simulink library "ESSLibrary"  (R2020a)
settings: Solver=VariableStepAuto  StartTime=0.0  StopTime=10.0  RelTol=1e-3
libraries: $bdroot x82, powerlib_meascontrol x10, simulink x7
(part 4 of 7)

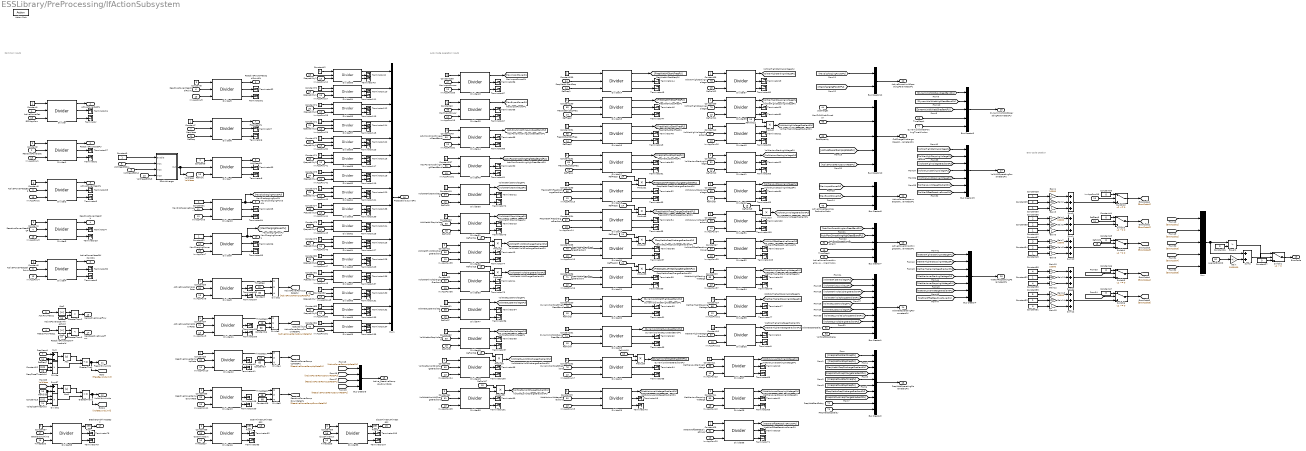
== system ESSLibrary/PreProcessing/IfActionSubsystem ==
  note: Error code creation
  note: Auto mode operation inputs
  note: Common inputs
  ActivePowerSet : Inport
  "ReactivePowerSet " : Inport  Port=2
  ActivePowerMeasECP : Inport  Port=3
  ReactivePowerMeasECP : Inport  Port=4
  ActivePowerMeasCtrlPoint : Inport  Port=5
  ReactivePowerMeasCtrlPoint : Inport  Port=6
  FreqMeas : Inport  Port=7
  VoltMeasECPL1 : Inport  Port=8
  VoltMeasECPL2 : Inport  Port=9
  VoltMeasECPL3 : Inport  Port=10
  MaxDischargingPower : Inport  Port=11
  MaxChargingPower : Inport  Port=12
  ECPAppPow : Inport  Port=13
  RefFreq : Inport  Port=14
  RefVolt : Inport  Port=15
  TimeStep : Inport  Port=16
  BreakerCmdTime : Inport  Port=17
  OpenTimeOut : Inport  Port=18
  CloseTimeOut : Inport  Port=19
  ActivePowerRampUpRate : Inport  Port=20
  ActivePowerRampDownRate : Inport  Port=21
  ReactivePowerRampUpRate : Inport  Port=22
  ReactivePowerRampDownRate : Inport  Port=23
  VoltCloseThreshold : Inport  Port=24
  FreqCloseThreshold : Inport  Port=25
  ActivePowerOpenThreshold : Inport  Port=26
  ReactivePowerOpenThreshold : Inport  Port=27
  Pcapability1 : Inport  Port=28
  Qcapability1 : Inport  Port=29
  Pcapability2 : Inport  Port=30
  Qcapability2 : Inport  Port=31
  Pcapability3 : Inport  Port=32
  Qcapability3 : Inport  Port=33
  Pcapability4 : Inport  Port=34
  Qcapability4 : Inport  Port=35
  Pcapability5 : Inport  Port=36
  Qcapability5 : Inport  Port=37
  Pcapability6 : Inport  Port=38
  Qcapability6 : Inport  Port=39
  Pcapability7 : Inport  Port=40
  Qcapability7 : Inport  Port=41
  Pcapability8 : Inport  Port=42
  Qcapability8 : Inport  Port=43
  SoCTarget : Inport  Port=44
  MaxChOrDischDuration : Inport  Port=45
  BattCapacity : Inport  Port=46
  MaxImportPower : Inport  Port=47
  MaxExportPower : Inport  Port=48
  ActivePowerReponseReductionRatio : Inport  Port=49
  ActvPowSmoothingLowDeadBand : Inport  Port=50
  ActvPowSmoothingHighDeadBand : Inport  Port=51
  ActvPowSmoothingGradient : Inport  Port=52
  ActivePowerSmoothingMovAvgTimeWindow : Inport  Port=53
  VoltWattHiStartVoltage : Inport  Port=54
  VoltWattHiStopVoltage : Inport  Port=55
  VoltWattHiVoltDischargeGradient : Inport  Port=56
  VoltWattHiVoltChargeGradient : Inport  Port=57
  VoltWattLoStartVoltage : Inport  Port=58
  VoltWattLoStopVoltage : Inport  Port=59
  VoltWattLoVoltDischargeGradient : Inport  Port=60
  VoltWattHLoVoltChargeGradient : Inport  Port=61
  VoltWattStartDelay : Inport  Port=62
  VoltWattStopDelay : Inport  Port=63
  FreqWattHiStartFreq : Inport  Port=64
  FreqWattHiStopFreq : Inport  Port=65
  FreqWattHiFreqDischargeGradient : Inport  Port=66
  FreqWattHiFreqChargeGradient : Inport  Port=67
  FreqWattLoStartFreq : Inport  Port=68
  FreqWattLoStopFreq : Inport  Port=69
  FreqWattLoFreqDischargeGradient : Inport  Port=70
  FreqWattLoFreqChargeGradient : Inport  Port=71
  FreqWattStartDelay : Inport  Port=72
  FreqWattStopDelay : Inport  Port=73
  DynamicVoltWattLowDeadBand : Inport  Port=74
  DynamicVoltWattHighDeadBand : Inport  Port=75
  DynamicVoltWattGradient : Inport  Port=76
  DynamicVoltWattMovAvgTimeWindow : Inport  Port=77
  VoltVarHighStartingVoltage : Inport  Port=78
  VoltVarHighStoppingVoltage : Inport  Port=79
  VoltVarHighVoltageGradient : Inport  Port=80
  VoltVarLowStartingVoltage : Inport  Port=81
  VoltVarLowStoppingVoltage : Inport  Port=82
  VoltVarLowVoltageGradient : Inport  Port=83
  VoltVarOffsetReactivePower : Inport  Port=84
  WattVarHighStartingWattage : Inport  Port=85
  WattVarHighStoppingWattage : Inport  Port=86
  WattVarHighWattageGradient : Inport  Port=87
  WattVarLowStartingWattage : Inport  Port=88
  WattVarLowStoppingWattage : Inport  Port=89
  WattVarLowWattageGradient : Inport  Port=90
  WattVarOffsetReactivePower : Inport  Port=91
  LogicalBlockID : Inport  Port=92  OutDataTypeStr=int32
  Action Port : ActionPort
  3PointAverge : MATLAB Function  TreatAsAtomicUnit=on
  Abs{,1..3} (4 alike) : Abs
  ActvPowMeas1 : InportShadow  Port=3
  Bus Creator1 : BusCreator  Inputs=10  OutDataTypeStr=Bus: VoltWattOperatingParametersPU
      settings: InheritFromInputs=off
  Bus Creator10 : BusCreator  Inputs=5  OutDataTypeStr=Bus: CrdChargeDischargeOperatingParametersPU
      settings: InheritFromInputs=off
  Bus Creator12 : BusCreator  Inputs=2  OutDataTypeStr=Bus: ActivePowerLimitOperatingParametersPU
      settings: InheritFromInputs=off
  Bus Creator19 : BusCreator  Inputs=7  OutDataTypeStr=Bus: VoltVarOperatingParametersPU
      settings: InheritFromInputs=off
  Bus Creator2 : BusCreator  Inputs=10  OutDataTypeStr=Bus: FreqWattOperatingParametersPU
      settings: InheritFromInputs=off
  Bus Creator3 : BusCreator  Inputs=5  OutDataTypeStr=Bus: DynamicVoltWattOperatingParameters
      settings: InheritFromInputs=off
  Bus Creator4 : BusCreator  Inputs=7  OutDataTypeStr=Bus: WattVarOperatingParametersPU
      settings: InheritFromInputs=off
  Bus Creator5 : BusCreator  Inputs=4  OutDataTypeStr=Bus: Active_ReactiveRampUp_DownData
      settings: InheritFromInputs=off
  Bus Creator7 : BusCreator  Inputs=5  OutDataTypeStr=Bus: ActivePowerSmoothingOperatingParametersPU
      settings: InheritFromInputs=off
  Bus Creator8 : BusCreator  Inputs=3  OutDataTypeStr=Bus: ActivePowerResponseOperatingParametersPU
      settings: InheritFromInputs=off
  Constant{,16..18} (4 alike) : Constant  Value=60  SampleTime=-1
  Constant{1..7,10..11,14..15,19..25,33..42,60..84,249..257,259..262,268} (67 alike) : Constant  OutDataTypeStr=boolean
  Constant12 : Constant  Value=0.01  SampleTime=-1
  Constant13 : Constant  Value=0.01  SampleTime=-1
  Constant{26..27,43..47} (7 alike) : Constant  Value=0  OutDataTypeStr=int64
  Constant{28,30,48..49,52..53} (6 alike) : Constant  OutDataTypeStr=int64
  Constant{29,54..56} (4 alike) : Constant  Value=2  OutDataTypeStr=int64
  Constant{8..9,31..32} (4 alike) : Constant  OutDataTypeStr=boolean  SampleTime=-1
  Constant50 : Constant  Value=4  OutDataTypeStr=int64
  Constant51 : Constant  Value=4  OutDataTypeStr=int64
  Constant57 : Constant  Value=3  OutDataTypeStr=int64
  Constant58 : Constant  Value=4  OutDataTypeStr=int64
  Constant59 : Constant  Value=5  OutDataTypeStr=int64
  Divide : Product  Inputs=***
  Divide1 : Product  Inputs=***
  Divide{2..5} (4 alike) : Product  Inputs=**/
  Divider{,1..69} (70 alike) : $bdroot/Divider  SystemSampleTime=-1  Latency=0  AutoFrameSizeCalculation=off
  Equal2 : RelationalOperator  Operator=>  OutDataTypeStr=boolean  RndMeth=Simplest
  Floor : Rounding  Operator=ceil
  Floor1 : Rounding  Operator=ceil
  Floor2 : Rounding  Operator=ceil
  FreqMeas1 : InportShadow  Port=7
  Gain : Gain  Gain=1000000
  Gain{1,4,7,10,13} (5 alike) : Gain  Gain=10000
  Gain{2,5,8,11,14} (5 alike) : Gain  Gain=100
  Gain{3,6,9,12,15} (5 alike) : Gain
  GreaterThan : RelationalOperator  Operator=<=  OutDataTypeStr=boolean  RndMeth=Simplest
  GreaterThan1 : RelationalOperator  Operator=<=  OutDataTypeStr=boolean  RndMeth=Simplest
  GreaterThan2 : RelationalOperator  Operator=<  OutDataTypeStr=boolean  RndMeth=Simplest
  GreaterThan3 : RelationalOperator  Operator=<  OutDataTypeStr=boolean  RndMeth=Simplest
  InvAppPow{1..51} (51 alike) : InportShadow  Port=13
  Mux : Mux  Inputs=5
  Mux1 : Mux  Inputs=16
  Product{,1..10} (11 alike) : Product
  ReactvPowMeas1 : InportShadow  Port=4
  RefFreq{1..10} (10 alike) : InportShadow  Port=14
  RefVolt{1..19} (19 alike) : InportShadow  Port=15
  Sum : Sum  Inputs=+-
  Sum{1,9..12} (5 alike) : Sum  Inputs=+++
  Sum2 : Sum  OutDataTypeStr=int64
  Sum87 : Sum  Inputs=+-
  Switch1 : Switch  Criteria=u2 > Threshold
  Switch{3..6,12} (5 alike) : Switch  Criteria=u2 ~= 0
  Terminator{,1..139} (140 alike) : Terminator
  TimeStep{1..8} (8 alike) : InportShadow  Port=16
  ActivePowerSetPU : Outport
  "ReactivePowerSetPU " : Outport  Port=2
  ActivePowerMeasPU : Outport  Port=3
  ReactivePowerMeasPU : Outport  Port=4
  ActivePowerMeasCtrlPointPU : Outport  Port=5
  ReactivePowerMeasCtrlPointPU : Outport  Port=6
  FreqMeasPU : Outport  Port=7
  VoltMeasPU : Outport  Port=8
  MaxDischargingPowerPU : Outport  Port=9
  MaxChargingPowerPU : Outport  Port=10
  FreqWithinLimits : Outport  Port=11
  VoltWithinLimits : Outport  Port=12
  ZeroActivePowerFlow : Outport  Port=13
  ZeroReactivePowerFlow : Outport  Port=14
  Active_ReactiveRampUp_DownData : Outport  Port=15  OutDataTypeStr=Bus: Active_ReactiveRampUp_DownData
  PQCapabiltyCurvePU : Outport  Port=16  OutDataTypeStr=double
  BreakerCmdTimeSteps : Outport  Port=17
  OpenTimeOutTimeSteps : Outport  Port=18
  CloseTimeOutTimeSteps : Outport  Port=19
  ActivePowerLimitOperatingParametersPU : Outport  Port=20  OutDataTypeStr=Bus: ActivePowerLimitOperatingParametersPU
  CrdChargeDischargeOperatingParametersPU : Outport  Port=21  OutDataTypeStr=Bus: CrdChargeDischargeOperatingParametersPU
  ActivePowerResponseOperatingParametersPU : Outport  Port=22  OutDataTypeStr=Bus: ActivePowerResponseOperatingParametersPU
  ActivePowerSmoothingOperatingParametersPU : Outport  Port=23  OutDataTypeStr=Bus: ActivePowerSmoothingOperatingParametersPU
  VoltWattOperatingParametersPU : Outport  Port=24  OutDataTypeStr=Bus: VoltWattOperatingParametersPU
  FreqWattOperatingParametersPU : Outport  Port=25  OutDataTypeStr=Bus: FreqWattOperatingParametersPU
  DynamicVoltWattOperatingParametersPU : Outport  Port=26  OutDataTypeStr=Bus: DynamicVoltWattOperatingParameters
  VoltVAROperatingParametersPU : Outport  Port=27  OutDataTypeStr=Bus: VoltVarOperatingParametersPU
  WattVAROperatingParametersPU : Outport  Port=28  OutDataTypeStr=Bus: WattVarOperatingParametersPU
  ErrorCode : Outport  Port=29
  tag scope: VoltMeas=global
  wires:
  VoltMeasECPL2/1 -> 3PointAverge/3(Inp2)
  VoltMeasECPL3/1 -> 3PointAverge/4(Inp3)
  RefVolt/1 -> Divider7/3
  Divider/1 -> ActivePowerSetPU/1
  Divider/3 -> Terminator/1
  Divider1/1 -> "ReactivePowerSetPU "/1
  RefFreq/1 -> Divider6/3
  InvAppPow1/1 -> Divider1/3
  InvAppPow2/1 -> Divider2/3
  InvAppPow3/1 -> Divider3/3
  Divider2/1 -> ActivePowerMeasPU/1
  Divider3/1 -> ReactivePowerMeasPU/1
  Divider4/1 -> ActivePowerMeasCtrlPointPU/1
  Divider5/1 -> ReactivePowerMeasCtrlPointPU/1
  Divider6/1 -> FreqMeasPU/1
  Divider7/1 -> VoltMeasPU/1
  [ErrorCode1] -> Mux/1
  [ErrorCode2] -> Mux/2
  [ErrorCode3] -> Mux/3
  [ErrorCode4] -> Mux/4
  [ErrorCode5] -> Mux/5
  Constant31/1 -> Divider10/1
  Constant32/1 -> Divider9/1
  MaxDischargingPower/1 -> Divider10/2
  VoltMeasECPL1/1 -> 3PointAverge/2(Inp1)
  Bus Creator5/1 -> Active_ReactiveRampUp_DownData/1
  [ActivePowerRampUpRatePU] -> Bus Creator5/1
  [ActivePowerRampDownRatePU] -> Bus Creator5/2
  [ReactivePowerRampUpRatePU] -> Bus Creator5/3
  [ReactivePowerRampDownRatePU] -> Bus Creator5/4
  Bus Creator2/1 -> FreqWattOperatingParametersPU/1
  Bus Creator3/1 -> DynamicVoltWattOperatingParametersPU/1
  Bus Creator1/1 -> VoltWattOperatingParametersPU/1
  Bus Creator7/1 -> ActivePowerSmoothingOperatingParametersPU/1
  Bus Creator8/1 -> ActivePowerResponseOperatingParametersPU/1
  Bus Creator12/1 -> ActivePowerLimitOperatingParametersPU/1
  Bus Creator10/1 -> CrdChargeDischargeOperatingParametersPU/1
  Bus Creator4/1 -> WattVAROperatingParametersPU/1
  Bus Creator19/1 -> VoltVAROperatingParametersPU/1
  InvAppPow32/1 -> Divider44/3
  Divider44/1 -> [ActvPowSmoothingLowDeadBandPU]
  Constant249/1 -> Divider44/1
  ActvPowSmoothingLowDeadBand/1 -> Divider44/2
  ActvPowSmoothingHighDeadBand/1 -> Divider45/2
  Constant257/1 -> Divider45/1
  Divider45/1 -> [ActvPowSmoothingHighDeadBandPU]
  InvAppPow31/1 -> Divider45/3
  Constant259/1 -> Divider14/1
  Divider14/1 -> [FreqWattHiStartFreqPU]
  RefFreq1/1 -> Divider14/3
  FreqWattHiStartFreq/1 -> Divider14/2
  FreqWattHiStopFreq/1 -> Divider15/2
  RefFreq2/1 -> Divider15/3
  Divider15/1 -> [FreqWattHiStopFreqPU]
  Constant250/1 -> Divider15/1
  Constant251/1 -> Divider16/1
  Divider16/1 -> [FreqWattLoStartFreqPU]
  RefFreq3/1 -> Divider16/3
  FreqWattLoStartFreq/1 -> Divider16/2
  Constant252/1 -> Divider17/1
  Divider17/1 -> [FreqWattLoStopFreqPU]
  FreqWattLoStopFreq/1 -> Divider17/2
  Constant253/1 -> Divider18/1
  InvAppPow13/1 -> Divider18/3
  FreqWattHiFreqDischargeGradient/1 -> Divider18/2
  InvAppPow14/1 -> Divider19/3
  FreqWattHiFreqChargeGradient/1 -> Divider19/2
  Constant254/1 -> Divider19/1
  FreqWattLoFreqDischargeGradient/1 -> Divider20/2
  InvAppPow15/1 -> Divider20/3
  Constant255/1 -> Divider20/1
  FreqWattLoFreqChargeGradient/1 -> Divider21/2
  InvAppPow16/1 -> Divider21/3
  Constant256/1 -> Divider21/1
  [FreqWattHiStartFreqPU] -> Bus Creator2/1
  [FreqWattHiStopFreqPU] -> Bus Creator2/2
  [FreqWattHiFreqDischargeGradientPU] -> Bus Creator2/3
  [FreqWattHiFreqChargeGradientPU] -> Bus Creator2/4
  [FreqWattLoStartFreqPU] -> Bus Creator2/5
  [FreqWattLoStopFreqPU] -> Bus Creator2/6
  [FreqWattLoFreqDischargeGradientPU] -> Bus Creator2/7
  [FreqWattLoFreqChargeGradientPU] -> Bus Creator2/8
  Constant260/1 -> Divider22/1
  RefVolt3/1 -> Divider22/3
  DynamicVoltWattHighDeadBand/1 -> Divider22/2
  Divider22/1 -> [DynamicVoltWattHighDeadBandPU]
  Divider23/1 -> [DynamicVoltWattLowDeadBandPU]
  DynamicVoltWattLowDeadBand/1 -> Divider23/2
  RefVolt4/1 -> Divider23/3
  Constant261/1 -> Divider23/1
  Constant262/1 -> Divider24/1
  InvAppPow17/1 -> Divider24/3
  DynamicVoltWattGradient/1 -> Divider24/2
  Divider30/1 -> [VoltWattHiStartVoltagePU]
  [ActvPowSmoothingLowDeadBandPU] -> Bus Creator7/1
  [ActvPowSmoothingHighDeadBandPU] -> Bus Creator7/2
  ActvPowSmoothingGradient/1 -> Bus Creator7/3
  ActivePowerSmoothingMovAvgTimeWindow/1 -> Bus Creator7/5
  Constant268/1 -> Divider43/1
  InvAppPow33/1 -> Divider43/3
  MaxImportPower/1 -> Divider43/2
  Divider43/1 -> [MaxImportPowerPU]
  [MaxImportPowerPU] -> Bus Creator8/1
  ActivePowerReponseReductionRatio/1 -> Bus Creator8/3
  SoCTarget/1 -> Bus Creator10/1
  MaxChOrDischDuration/1 -> Bus Creator10/2
  Divider10/1 -> [MaxDischargingPowerPU], MaxDischargingPowerPU/1
  Divider9/1 -> [MaxChargingPowerPU], MaxChargingPowerPU/1
  [MaxDischargingPowerPU] -> Bus Creator12/1
  [MaxChargingPowerPU] -> Bus Creator12/2
  Divider37/1 -> [VoltVarHighStartingVoltagePU]
  ECPAppPow/1 -> Divider/3
  ActivePowerRampUpRate/1 -> Divider8/2
  ActivePowerRampDownRate/1 -> Divider11/2
  ReactivePowerRampUpRate/1 -> Divider12/2
  ReactivePowerRampDownRate/1 -> Divider13/2
  Constant33/1 -> Divider8/1
  Constant34/1 -> Divider11/1
  Constant35/1 -> Divider12/1
  Constant36/1 -> Divider13/1
  ActivePowerSet/1 -> Divider/2
  "ReactivePowerSet "/1 -> Divider1/2
  Constant1/1 -> Divider/1
  Constant2/1 -> Divider1/1
  ActivePowerMeasECP/1 -> Divider2/2
  Constant3/1 -> Divider2/1
  ReactivePowerMeasECP/1 -> Divider3/2
  Constant4/1 -> Divider3/1
  ActivePowerMeasCtrlPoint/1 -> Divider4/2
  Constant5/1 -> Divider4/1
  ReactivePowerMeasCtrlPoint/1 -> Divider5/2
  Constant6/1 -> Divider5/1
  FreqMeas/1 -> Divider6/2
  Constant7/1 -> Divider6/1
  Constant8/1 -> Divider7/1
  3PointAverge/1(Out) -> Divider7/2, [VoltMeas]
  Constant9/1 -> 3PointAverge/1(Enable)
  FreqMeas1/1 -> Sum/1
  RefFreq7/1 -> Divide/1, Sum/2
  Sum/1 -> Abs/1
  GreaterThan/1 -> FreqWithinLimits/1, [FreqBeyondLimit]
  Abs/1 -> GreaterThan/1
  Divide/1 -> GreaterThan/2
  Constant12/1 -> Divide/2
  FreqCloseThreshold/1 -> Divide/3
  VoltCloseThreshold/1 -> Divide1/3
  Constant13/1 -> Divide1/2
  Divide1/1 -> GreaterThan1/2
  Abs1/1 -> GreaterThan1/1
  GreaterThan1/1 -> [VoltBeyondLimit], VoltWithinLimits/1
  Sum87/1 -> Abs1/1
  Abs2/1 -> GreaterThan2/1
  ActvPowMeas1/1 -> Abs2/1
  ActivePowerOpenThreshold/1 -> GreaterThan2/2
  ReactvPowMeas1/1 -> Abs3/1
  Abs3/1 -> GreaterThan3/1
  ReactivePowerOpenThreshold/1 -> GreaterThan3/2
  GreaterThan3/1 -> ZeroReactivePowerFlow/1
  GreaterThan2/1 -> ZeroActivePowerFlow/1
  Divide2/1 -> [ActivePowerRampUpRatePU]
  Divider8/1 -> Divide2/1
  TimeStep/1 -> Divide2/2
  Constant/1 -> Divide2/3
  TimeStep1/1 -> Divide3/2
  Constant16/1 -> Divide3/3
  Divider11/1 -> Divide3/1
  Divide3/1 -> [ActivePowerRampDownRatePU]
  Divide4/1 -> [ReactivePowerRampUpRatePU]
  Divider12/1 -> Divide4/1
  Constant17/1 -> Divide4/3
  TimeStep2/1 -> Divide4/2
  Constant18/1 -> Divide5/3
  Divider13/1 -> Divide5/1
  TimeStep3/1 -> Divide5/2
  Divide5/1 -> [ReactivePowerRampDownRatePU]
  InvAppPow36/1 -> Divider33/3
  Constant22/1 -> Divider33/1
  Divider33/2 -> Terminator14/1
  Divider32/2 -> Terminator13/1
  Constant21/1 -> Divider32/1
  InvAppPow35/1 -> Divider32/3
  Divider31/1 -> [VoltWattHiStopVoltagePU]
  RefVolt2/1 -> Divider31/3
  Constant20/1 -> Divider31/1
  Divider30/2 -> Terminator12/1
  Constant19/1 -> Divider30/1
  RefVolt1/1 -> Divider30/3
  VoltWattHiStartVoltage/1 -> Divider30/2
  VoltWattHiStopVoltage/1 -> Divider31/2
  VoltWattHiVoltDischargeGradient/1 -> Divider32/2
  VoltWattHiVoltChargeGradient/1 -> Divider33/2
  WattVarHighStoppingWattage/1 -> Divider35/2
  InvAppPow21/1 -> Divider35/3
  Constant24/1 -> Divider35/1
  Divider35/2 -> Terminator17/1
  Divider37/2 -> Terminator19/1
  Constant38/1 -> Divider37/1
  RefVolt12/1 -> Divider37/3
  WattVarHighStartingWattage/1 -> Divider34/2
  InvAppPow37/1 -> Divider34/3
  Constant23/1 -> Divider34/1
  Divider34/2 -> Terminator16/1
  Divider35/1 -> [WattVarHigherStoppingWattagePU]
  Divider34/1 -> [WattVarHigherStartingWattagePU]
  VoltVarHighStartingVoltage/1 -> Divider37/2
  InvAppPow26/1 -> Divider40/3
  Constant39/1 -> Divider39/1
  Constant40/1 -> Divider40/1
  Divider39/2 -> Terminator23/1
  RefVolt11/1 -> Divider39/3
  Divider41/2 -> Terminator22/1
  Divider39/1 -> [VoltVarHighStoppingVoltagePU]
  RefVolt10/1 -> Divider41/3
  Divider40/2 -> Terminator21/1
  Constant41/1 -> Divider41/1
  VoltVarHighStoppingVoltage/1 -> Divider39/2
  VoltVarHighVoltageGradient/1 -> Divider40/2
  VoltVarLowStartingVoltage/1 -> Divider41/2
  [DynamicVoltWattGradientPU] -> Bus Creator3/3
  TimeStep4/1 -> Bus Creator3/4
  DynamicVoltWattMovAvgTimeWindow/1 -> Bus Creator3/5
  Constant42/1 -> Divider55/1
  Gain1/1 -> Sum9/1
  Gain2/1 -> Sum9/2
  Gain3/1 -> Sum9/3
  Switch12/1 -> [ErrorCode1]
  InvAppPow38/1 -> Switch12/2
  Sum9/1 -> Switch12/3
  Constant43/1 -> Switch12/1
  Constant44/1 -> Switch3/1
  Sum1/1 -> Switch3/3
  RefFreq8/1 -> Switch3/2
  Switch3/1 -> [ErrorCode2]
  Switch4/1 -> [ErrorCode3]
  RefVolt6/1 -> Switch4/2
  Sum10/1 -> Switch4/3
  Constant45/1 -> Switch4/1
  [FreqBeyondLimit] -> Switch5/2
  Sum11/1 -> Switch5/3
  [VoltBeyondLimit] -> Switch6/2
  Sum12/1 -> Switch6/3
  Switch5/1 -> [ErrorCode4]
  Switch6/1 -> [ErrorCode5]
  Divider/2 -> Terminator24/1
  Divider1/2 -> Terminator27/1
  Divider1/3 -> Terminator2/1
  Divider2/3 -> Terminator3/1
  Divider2/2 -> Terminator28/1
  Divider3/2 -> Terminator4/1
  Divider3/3 -> Terminator29/1
  InvAppPow4/1 -> Divider4/3
  Divider4/3 -> Terminator5/1
  Divider4/2 -> Terminator30/1
  InvAppPow5/1 -> Divider5/3
  Divider6/2 -> Terminator7/1
  Divider6/3 -> Terminator6/1
  Divider5/2 -> Terminator32/1
  Divider5/3 -> Terminator31/1
  Divider7/3 -> Terminator8/1
  Divider7/2 -> Terminator33/1
  InvAppPow6/1 -> Divider10/3
  Divider10/2 -> Terminator25/1
  Divider10/3 -> Terminator34/1
  MaxChargingPower/1 -> Divider9/2
  InvAppPow7/1 -> Divider9/3
  Divider9/3 -> Terminator35/1
  Divider9/2 -> Terminator26/1
  InvAppPow8/1 -> Divider8/3
  Divider8/3 -> Terminator37/1
  Divider8/2 -> Terminator36/1
  InvAppPow9/1 -> Divider11/3
  Divider11/3 -> Terminator39/1
  Divider11/2 -> Terminator38/1
  InvAppPow10/1 -> Divider12/3
  Divider12/2 -> Terminator40/1
  Divider12/3 -> Terminator41/1
  InvAppPow11/1 -> Divider13/3
  Divider55/2 -> Terminator42/1
  Divider55/3 -> Terminator43/1
  InvAppPow12/1 -> Divider55/3
  RefFreq4/1 -> Divider17/3
  Divider31/2 -> Terminator15/1
  Sum2/1 -> Switch1/1
  Constant26/1 -> Equal2/2
  Equal2/1 -> Switch1/2
  LogicalBlockID/1 -> Gain/1
  Mux/1 -> Sum2/1, Equal2/1
  Switch1/1 -> ErrorCode/1
  Constant27/1 -> Switch1/3
  Gain/1 -> Sum2/2
  Gain6/1 -> Sum1/3
  Gain5/1 -> Sum1/2
  Gain4/1 -> Sum1/1
  Gain7/1 -> Sum10/1
  Gain8/1 -> Sum10/2
  Gain9/1 -> Sum10/3
  Gain12/1 -> Sum11/3
  Gain11/1 -> Sum11/2
  Gain10/1 -> Sum11/1
  Gain13/1 -> Sum12/1
  Gain14/1 -> Sum12/2
  Gain15/1 -> Sum12/3
  Constant28/1 -> Gain1/1
  Constant29/1 -> Gain2/1
  Constant30/1 -> Gain3/1
  Constant48/1 -> Gain6/1
  Constant49/1 -> Gain9/1
  Constant50/1 -> Gain12/1
  Constant51/1 -> Gain15/1
  Constant52/1 -> Gain11/1
  Constant53/1 -> Gain14/1
  Constant54/1 -> Gain8/1
  Constant55/1 -> Gain5/1
  Constant56/1 -> Gain4/1
  Constant57/1 -> Gain7/1
  Constant58/1 -> Gain10/1
  Constant59/1 -> Gain13/1
  Divider14/2 -> Terminator44/1
  Divider14/3 -> Terminator45/1
  Divider15/2 -> Terminator46/1
  Divider15/3 -> Terminator47/1
  Divider16/2 -> Terminator48/1
  Divider16/3 -> Terminator49/1
  Divider17/2 -> Terminator50/1
  Divider17/3 -> Terminator51/1
  Divider18/2 -> Terminator52/1
  Divider18/3 -> Terminator53/1
  Divider19/2 -> Terminator54/1
  Divider19/3 -> Terminator55/1
  Divider20/2 -> Terminator56/1
  Divider20/3 -> Terminator57/1
  Divider21/2 -> Terminator58/1
  Divider21/3 -> Terminator59/1
  Divider22/2 -> Terminator60/1
  Divider22/3 -> Terminator61/1
  Divider23/2 -> Terminator62/1
  Divider23/3 -> Terminator63/1
  Divider24/2 -> Terminator64/1
  Divider24/3 -> Terminator65/1
  Divider30/3 -> Terminator72/1
  Divider31/3 -> Terminator73/1
  Divider32/3 -> Terminator74/1
  Divider33/3 -> Terminator75/1
  Divider34/3 -> Terminator76/1
  Divider35/3 -> Terminator77/1
  Divider37/3 -> Terminator80/1
  Divider39/3 -> Terminator81/1
  Divider40/3 -> Terminator82/1
  Divider41/3 -> Terminator83/1
  Divider43/2 -> Terminator86/1
  Divider43/3 -> Terminator87/1
  Divider44/3 -> Terminator89/1
  Divider44/2 -> Terminator88/1
  Divider45/2 -> Terminator90/1
  Divider45/3 -> Terminator91/1
  RefVolt5/1 -> Divide1/1, Sum87/2
  [VoltMeas] -> Sum87/1
  FreqWattStartDelay/1 -> Bus Creator2/9
  FreqWattStopDelay/1 -> Bus Creator2/10
  [DynamicVoltWattLowDeadBandPU] -> Bus Creator3/1
  [DynamicVoltWattHighDeadBandPU] -> Bus Creator3/2
  Divider25/3 -> Terminator67/1
  Divider25/2 -> Terminator66/1
  Divider25/1 -> [MaxExportPowerPU]
  MaxExportPower/1 -> Divider25/2
  InvAppPow18/1 -> Divider25/3
  Constant60/1 -> Divider25/1
  [MaxExportPowerPU] -> Bus Creator8/2
  BattCapacity/1 -> Bus Creator10/3
  [ActivePowerRampUpRatePU] -> Bus Creator10/4
  [ActivePowerRampDownRatePU] -> Bus Creator10/5
  TimeStep5/1 -> Bus Creator7/4
  VoltWattLoStopVoltage/1 -> Divider48/2
  Divider48/2 -> Terminator95/1
  Divider48/3 -> Terminator97/1
  Constant61/1 -> Divider47/1
  Divider48/1 -> [VoltWattLoStopVoltagePU]
  Divider47/3 -> Terminator96/1
  RefVolt8/1 -> Divider48/3
  Constant62/1 -> Divider48/1
  RefVolt7/1 -> Divider47/3
  Divider47/1 -> [VoltWattLoStartVoltagePU]
  Divider47/2 -> Terminator94/1
  VoltWattLoStartVoltage/1 -> Divider47/2
  Divider50/3 -> Terminator101/1
  Divider49/3 -> Terminator100/1
  VoltWattHLoVoltChargeGradient/1 -> Divider50/2
  VoltWattLoVoltDischargeGradient/1 -> Divider49/2
  InvAppPow24/1 -> Divider49/3
  Constant63/1 -> Divider49/1
  Divider49/2 -> Terminator98/1
  Divider50/2 -> Terminator99/1
  Constant64/1 -> Divider50/1
  InvAppPow25/1 -> Divider50/3
  [VoltWattHiStartVoltagePU] -> Bus Creator1/1
  [VoltWattHiStopVoltagePU] -> Bus Creator1/2
  [VoltWattHiVoltDischargeGradientPU] -> Bus Creator1/3
  [VoltWattHiVoltChargeGradientPU] -> Bus Creator1/4
  [VoltWattLoStartVoltagePU] -> Bus Creator1/5
  [VoltWattLoStopVoltagePU] -> Bus Creator1/6
  [VoltWattLLoVoltDischargeGradientPU] -> Bus Creator1/7
  [VoltWattLoVoltChargeGradientPU] -> Bus Creator1/8
  VoltWattStartDelay/1 -> Bus Creator1/9
  VoltWattStopDelay/1 -> Bus Creator1/10
  Constant65/1 -> Divider42/1
  VoltVarLowStoppingVoltage/1 -> Divider42/2
  RefVolt9/1 -> Divider42/3
  Divider42/1 -> [VoltVarLowStoppingVoltagePU]
  Divider42/3 -> Terminator85/1
  Divider42/2 -> Terminator84/1
  Constant66/1 -> Divider51/1
  VoltVarLowVoltageGradient/1 -> Divider51/2
  InvAppPow34/1 -> Divider51/3
  Divider51/2 -> Terminator102/1
  Divider51/3 -> Terminator103/1
  Constant67/1 -> Divider52/1
  VoltVarOffsetReactivePower/1 -> Divider52/2
  InvAppPow39/1 -> Divider52/3
  Divider52/1 -> [VoltVarOffsetReactivePowerPU]
  Divider52/2 -> Terminator104/1
  Divider52/3 -> Terminator105/1
  [VoltVarOffsetReactivePowerPU] -> Bus Creator19/7
  [VoltVarLowVoltageGradientPU] -> Bus Creator19/6
  [VoltVarLowStoppingVoltagePU] -> Bus Creator19/5
  [VoltVarLowStartingVoltagePU] -> Bus Creator19/4
  [VoltVarHighVoltageGradientPU] -> Bus Creator19/3
  [VoltVarHighStoppingVoltagePU] -> Bus Creator19/2
  [VoltVarHighStartingVoltagePU] -> Bus Creator19/1
  Divider26/3 -> Terminator9/1
  Divider26/2 -> Terminator1/1
  Constant10/1 -> Divider26/1
  InvAppPow22/1 -> Divider26/3
  WattVarHighWattageGradient/1 -> Divider26/2
  Divider26/1 -> [WattVarHigherWattageGradientPU]
  Divider28/3 -> Terminator69/1
  Divider27/3 -> Terminator68/1
  Divider27/1 -> [WattVarLowerStartingWattagePU]
  Divider28/1 -> [WattVarLowerStoppingWattagePU]
  Divider27/2 -> Terminator10/1
  Constant11/1 -> Divider27/1
  Divider28/2 -> Terminator11/1
  Constant14/1 -> Divider28/1
  WattVarLowStartingWattage/1 -> Divider27/2
  WattVarLowStoppingWattage/1 -> Divider28/2
  InvAppPow23/1 -> Divider27/3
  InvAppPow40/1 -> Divider28/3
  Constant25/1 -> Divider36/1
  Divider36/2 -> Terminator20/1
  Constant15/1 -> Divider29/1
  Divider29/2 -> Terminator18/1
  Divider36/1 -> [WattVarOffsetReactivePowerPU]
  Divider29/1 -> [WattVarLowerWattageGradientPU]
  Divider29/3 -> Terminator70/1
  Divider36/3 -> Terminator71/1
  WattVarLowWattageGradient/1 -> Divider29/2
  WattVarOffsetReactivePower/1 -> Divider36/2
  InvAppPow19/1 -> Divider29/3
  InvAppPow20/1 -> Divider36/3
  [WattVarHigherStartingWattagePU] -> Bus Creator4/1
  [WattVarHigherStoppingWattagePU] -> Bus Creator4/2
  [WattVarHigherWattageGradientPU] -> Bus Creator4/3
  [WattVarLowerStartingWattagePU] -> Bus Creator4/4
  [WattVarLowerStoppingWattagePU] -> Bus Creator4/5
  [WattVarLowerWattageGradientPU] -> Bus Creator4/6
  [WattVarOffsetReactivePowerPU] -> Bus Creator4/7
  Product/1 -> [VoltVarHighVoltageGradientPU]
  Divider41/1 -> [VoltVarLowStartingVoltagePU]
  Divider40/1 -> Product/2
  RefVolt13/1 -> Product/1
  Constant46/1 -> Switch5/1
  Constant47/1 -> Switch6/1
  Divider32/1 -> Product2/2
  Product2/1 -> [VoltWattHiVoltDischargeGradientPU]
  RefVolt14/1 -> Product2/1
  Divider33/1 -> Product3/2
  Product3/1 -> [VoltWattHiVoltChargeGradientPU]
  RefVolt15/1 -> Product3/1
  Product4/1 -> [VoltWattLLoVoltDischargeGradientPU]
  Divider49/1 -> Product4/2
  RefVolt16/1 -> Product4/1
  Product5/1 -> [VoltWattLoVoltChargeGradientPU]
  Divider50/1 -> Product5/2
  RefVolt17/1 -> Product5/1
  Divider18/1 -> Product1/2
  Product1/1 -> [FreqWattHiFreqDischargeGradientPU]
  RefFreq5/1 -> Product1/1
  Divider19/1 -> Product6/2
  Product6/1 -> [FreqWattHiFreqChargeGradientPU]
  RefFreq6/1 -> Product6/1
  Divider20/1 -> Product7/2
  Product7/1 -> [FreqWattLoFreqDischargeGradientPU]
  RefFreq9/1 -> Product7/1
  Divider21/1 -> Product8/2
  Product8/1 -> [FreqWattLoFreqChargeGradientPU]
  RefFreq10/1 -> Product8/1
  Product9/1 -> [DynamicVoltWattGradientPU]
  Divider24/1 -> Product9/2
  RefVolt18/1 -> Product9/1
  Divider51/1 -> Product10/2
  Product10/1 -> [VoltVarLowVoltageGradientPU]
  RefVolt19/1 -> Product10/1
  Constant37/1 -> Divider38/1
  Constant68/1 -> Divider46/1
  Constant69/1 -> Divider53/1
  BreakerCmdTime/1 -> Divider38/2
  OpenTimeOut/1 -> Divider46/2
  CloseTimeOut/1 -> Divider53/2
  TimeStep6/1 -> Divider38/3
  TimeStep7/1 -> Divider46/3
  TimeStep8/1 -> Divider53/3
  Divider38/1 -> Floor/1
  Divider46/1 -> Floor1/1
  Divider53/1 -> Floor2/1
  Divider38/2 -> Terminator78/1
  Divider38/3 -> Terminator79/1
  Divider46/2 -> Terminator92/1
  Divider46/3 -> Terminator93/1
  Divider53/2 -> Terminator106/1
  Divider53/3 -> Terminator107/1
  Floor/1 -> BreakerCmdTimeSteps/1
  Floor1/1 -> OpenTimeOutTimeSteps/1
  Floor2/1 -> CloseTimeOutTimeSteps/1
  Divider13/2 -> Terminator108/1
  Divider13/3 -> Terminator109/1
  Pcapability1/1 -> Divider55/2
  Divider54/3 -> Terminator111/1
  Divider54/2 -> Terminator110/1
  Divider56/2 -> Terminator112/1
  Divider56/3 -> Terminator113/1
  Divider57/3 -> Terminator115/1
  Divider57/2 -> Terminator114/1
  Divider61/2 -> Terminator120/1
  Divider61/3 -> Terminator121/1
  Divider60/3 -> Terminator119/1
  Divider60/2 -> Terminator118/1
  Divider58/2 -> Terminator116/1
  Divider58/3 -> Terminator117/1
  Divider59/3 -> Terminator123/1
  Divider59/2 -> Terminator122/1
  Divider67/2 -> Terminator136/1
  Divider67/3 -> Terminator137/1
  Divider66/3 -> Terminator131/1
  Divider66/2 -> Terminator130/1
  Divider68/2 -> Terminator132/1
  Divider68/3 -> Terminator133/1
  Divider69/3 -> Terminator135/1
  Divider69/2 -> Terminator134/1
  Divider65/2 -> Terminator128/1
  Divider65/3 -> Terminator129/1
  Divider64/3 -> Terminator127/1
  Divider64/2 -> Terminator126/1
  Divider62/2 -> Terminator124/1
  Divider62/3 -> Terminator125/1
  Divider63/3 -> Terminator139/1
  Divider63/2 -> Terminator138/1
  InvAppPow27/1 -> Divider54/3
  InvAppPow28/1 -> Divider56/3
  InvAppPow29/1 -> Divider57/3
  InvAppPow30/1 -> Divider59/3
  InvAppPow41/1 -> Divider58/3
  InvAppPow42/1 -> Divider60/3
  InvAppPow43/1 -> Divider61/3
  InvAppPow44/1 -> Divider63/3
  InvAppPow45/1 -> Divider62/3
  InvAppPow46/1 -> Divider64/3
  InvAppPow47/1 -> Divider65/3
  InvAppPow48/1 -> Divider67/3
  InvAppPow49/1 -> Divider66/3
  InvAppPow50/1 -> Divider68/3
  InvAppPow51/1 -> Divider69/3
  Qcapability1/1 -> Divider54/2
  Pcapability2/1 -> Divider56/2
  Qcapability2/1 -> Divider57/2
  Pcapability3/1 -> Divider59/2
  Qcapability3/1 -> Divider58/2
  Pcapability4/1 -> Divider60/2
  Qcapability4/1 -> Divider61/2
  Pcapability5/1 -> Divider63/2
  Qcapability5/1 -> Divider62/2
  Pcapability6/1 -> Divider64/2
  Qcapability6/1 -> Divider65/2
  Pcapability7/1 -> Divider67/2
  Qcapability7/1 -> Divider66/2
  Pcapability8/1 -> Divider68/2
  Qcapability8/1 -> Divider69/2
  Constant70/1 -> Divider54/1
  Constant71/1 -> Divider56/1
  Constant72/1 -> Divider57/1
  Constant73/1 -> Divider59/1
  Constant74/1 -> Divider58/1
  Constant75/1 -> Divider60/1
  Constant76/1 -> Divider61/1
  Constant77/1 -> Divider63/1
  Constant78/1 -> Divider62/1
  Constant79/1 -> Divider64/1
  Constant80/1 -> Divider65/1
  Constant81/1 -> Divider67/1
  Constant82/1 -> Divider66/1
  Constant83/1 -> Divider68/1
  Constant84/1 -> Divider69/1
  Mux1/1 -> PQCapabiltyCurvePU/1
  Divider55/1 -> Mux1/1
  Divider69/1 -> Mux1/16
  Divider54/1 -> Mux1/2
  Divider56/1 -> Mux1/3
  Divider57/1 -> Mux1/4
  Divider59/1 -> Mux1/5
  Divider58/1 -> Mux1/6
  Divider60/1 -> Mux1/7
  Divider61/1 -> Mux1/8
  Divider63/1 -> Mux1/9
  Divider62/1 -> Mux1/10
  Divider64/1 -> Mux1/11
  Divider65/1 -> Mux1/12
  Divider67/1 -> Mux1/13
  Divider66/1 -> Mux1/14
  Divider68/1 -> Mux1/15

== system ESSLibrary/QReference_PF/If Action Subsystem ==
  PFSet : Inport
  PFSign : Inport  Port=2
  PSet : Inport  Port=3
  Action Port : ActionPort
  Subsystem1 : Subsystem
  PFSetQSet : Outport
  ErrorCode : Outport  Port=2
  wires:
  PFSign/1 -> Subsystem1/2(PFSign)
  Subsystem1/1(QOut) -> PFSetQSet/1
  PFSet/1 -> Subsystem1/1(PF)
  PSet/1 -> Subsystem1/3(PMeas)
  Subsystem1/2(ErrorCode) -> ErrorCode/1

== system ESSLibrary/QReference_PF/If Action Subsystem1 ==
  Action Port : ActionPort
  Constant : Constant  Value=0  SampleTime=-1
  PFSetQSetPU : Outport
  ErrorCode : Outport  Port=2
  wires:
  Constant/1 -> PFSetQSetPU/1, ErrorCode/1

== system ESSLibrary/SoCManagement/ElseActionSubsystem ==
  Action Port : ActionPort
  Constant1 : Constant  Value=0  OutDataTypeStr=int64  SampleTime=-1
  Constant2 : Constant  Value=0  OutDataTypeStr=boolean
  Constant3 : Constant  Value=0  OutDataTypeStr=double
  SoCFinal : Outport  OutDataTypeStr=double
  SoCNextStep : Outport  Port=2  OutDataTypeStr=double
  ChargeEnable : Outport  Port=3  OutDataTypeStr=boolean
  DischargeEnable : Outport  Port=4  OutDataTypeStr=boolean
  ErrorCodeOut : Outport  Port=5  OutDataTypeStr=int64
  wires:
  Constant2/1 -> ChargeEnable/1, DischargeEnable/1
  Constant1/1 -> ErrorCodeOut/1
  Constant3/1 -> SoCNextStep/1, SoCFinal/1

== system ESSLibrary/SoCManagement/IfActionSubsystem ==
  ActivePowerMeasECP : Inport  OutDataTypeStr=double
  SoCMeas : Inport  Port=2  OutDataTypeStr=double
  SoCMin : Inport  Port=3
  SoCMax : Inport  Port=4
  BattCapacity : Inport  Port=5  OutDataTypeStr=double
  ECPAppPow : Inport  Port=6  OutDataTypeStr=double
  TimeStep : Inport  Port=7
  ActiveReactivePowerRampUpDownData : Inport  Port=8  OutDataTypeStr=Bus: ActiveReactiveRampUpDownData
  LogicalBlockID : Inport  Port=9  OutDataTypeStr=int64
  Action Port : ActionPort
  Bus Selector : BusSelector  OutputSignals=ActivePowerRampUpRatePU,ActivePowerRampDownRatePU
  Comparator : Subsystem
  Constant1 : Constant  OutDataTypeStr=boolean
  Constant10 : Constant  Value=0  OutDataTypeStr=int64
  Constant11 : Constant  Value=0  OutDataTypeStr=int64
  Constant12 : Constant  Value=2  OutDataTypeStr=int32
  Constant13 : Constant  Value=0.0  OutDataTypeStr=double
  Constant15 : Constant  Value=0.0  OutDataTypeStr=double
  Constant17 : Constant  OutDataTypeStr=int64
  Constant5 : Constant  Value=0  OutDataTypeStr=boolean
  Constant6 : Constant  OutDataTypeStr=boolean
  Constant7 : Constant  Value=0  OutDataTypeStr=boolean
  Constant8 : Constant  OutDataTypeStr=boolean
  Equal2 : RelationalOperator  Operator=>  OutDataTypeStr=boolean  RndMeth=Simplest
  Gain1 : Gain  Gain=1000000
  RemainingEnergyCalculator : MATLAB Function  TreatAsAtomicUnit=on
  Sum1 : Sum  OutDataTypeStr=int64
  Switch : Switch  Criteria=u2 ~= 0
  Switch1 : Switch  Criteria=u2 ~= 0
  Switch4 : Switch  Criteria=u2 > Threshold
  SoCFinal : Outport  OutDataTypeStr=double
  SoCNextStep : Outport  Port=2  OutDataTypeStr=double
  ChargeEnable : Outport  Port=3
  DischargeEnable : Outport  Port=4
  ErrorCodeOut : Outport  Port=5  OutDataTypeStr=int64
  wires:
  SoCMin/1 -> Comparator/4(LowerTrhd)
  Constant1/1 -> Comparator/1(Enable/Disable)
  SoCMax/1 -> Comparator/3(UpperTrhd)
  Constant12/1 -> Comparator/5(HystSelection)
  Constant13/1 -> Comparator/7(RelHyst)
  Constant17/1 -> Comparator/8(VariableIdentifier)
  Constant15/1 -> Comparator/6(AbsHyst)
  Constant6/1 -> Switch/3
  Constant7/1 -> Switch1/1
  Constant8/1 -> Switch1/3
  Constant5/1 -> Switch/1
  SoCMeas/1 -> RemainingEnergyCalculator/2(SoCMeas)
  BattCapacity/1 -> RemainingEnergyCalculator/3(BatteryCapacity)
  ECPAppPow/1 -> RemainingEnergyCalculator/4(BasePower)
  Bus Selector/1 -> RemainingEnergyCalculator/6(ActivePowerRampUpRate)  "<ActivePowerRampUpRatePU>"
  Bus Selector/2 -> RemainingEnergyCalculator/7(ActivePowerRampDownRate)  "<ActivePowerRampDownRatePU>"
  TimeStep/1 -> RemainingEnergyCalculator/5(TimeStep)
  ActivePowerMeasECP/1 -> RemainingEnergyCalculator/1(ActivePowerMeasPU)
  Switch/1 -> ChargeEnable/1
  Switch1/1 -> DischargeEnable/1
  RemainingEnergyCalculator/1(SoCFinal) -> Comparator/2("Input "), SoCFinal/1
  RemainingEnergyCalculator/2(SoCNextStep) -> SoCNextStep/1
  Comparator/2(MaxLimitCrossed) -> Switch/2
  Comparator/3(MinLimitCrossed) -> Switch1/2
  Gain1/1 -> Sum1/2
  Equal2/1 -> Switch4/2
  Constant11/1 -> Switch4/3
  Sum1/1 -> Switch4/1
  LogicalBlockID/1 -> Gain1/1
  Switch4/1 -> ErrorCodeOut/1
  Comparator/1(ErrorCode) -> Equal2/1, Sum1/1
  Constant10/1 -> Equal2/2
  ActiveReactivePowerRampUpDownData/1 -> Bus Selector/1

== system ESSLibrary/ActivePowerSmoothing/MovAvgDeltaVoltCalc/ElseMovAvgFilter ==
  Inp : Inport
  Action Port : ActionPort
  Constant : Constant  Value=0  OutDataTypeStr=int64  SampleTime=-1
  Out : Outport
  ErrorCode : Outport  Port=2
  wires:
  Inp/1 -> Out/1
  Constant/1 -> ErrorCode/1

== system ESSLibrary/ActivePowerSmoothing/MovAvgDeltaVoltCalc/IfMovAvgFilter ==
  Inp : Inport
  FilterTime : Inport  Port=2
  TimeStep : Inport  Port=3
  Action Port : ActionPort
  Constant : Constant  Value=0
  Constant1 : Constant  Value=0
  DiscreteMovingAverage : MATLAB Function  TreatAsAtomicUnit=on
  Enabled Subsystem : Subsystem  TreatAsAtomicUnit=on
  Relational Operator : RelationalOperator  Operator=>  OutDataTypeStr=boolean  ZeroCross=off  RndMeth=Simplest
  Switch : Switch  Criteria=u2 > Threshold
  Out : Outport
  ErrorCode : Outport  Port=2
  wires:
  Inp/1 -> DiscreteMovingAverage/2(Inp)
  Constant/1 -> Relational Operator/2
  FilterTime/1 -> Enabled Subsystem/2(FilterTime)
  Switch/1 -> DiscreteMovingAverage/1(NoOfTS)
  Enabled Subsystem/1(NoOfTimeStep) -> Switch/1
  Relational Operator/1 -> Switch/2, Enabled Subsystem/Enable
  TimeStep/1 -> Enabled Subsystem/1(TimeStep), Relational Operator/1
  DiscreteMovingAverage/1(Out) -> Out/1
  Constant1/1 -> Switch/3
  DiscreteMovingAverage/2(ErrorCode) -> ErrorCode/1

== system ESSLibrary/ChargeDischargeStorageMode/Comparator/Basic alarm ver2.0 ==
  Enable/disable : Inport  OutDataTypeStr=boolean
  "Input " : Inport  Port=2
  UpperTrhd : Inport  Port=3
  LowerTrhd : Inport  Port=4
  HystSelection : Inport  Port=5  OutDataTypeStr=int32
  AbsHyst : Inport  Port=6
  RelHyst : Inport  Port=7
  Enable/disable1 : InportShadow  OutDataTypeStr=boolean
  Enabled Subsystem : Subsystem  TreatAsAtomicUnit=on
  Enabled Subsystem1 : Subsystem  TreatAsAtomicUnit=on
  If : If  IfExpression=u1 ~=0
  Switch : Switch  Criteria=u2 > Threshold
  Switch1 : Switch  Criteria=u2 > Threshold
  Switch3 : Switch  Criteria=u2 > Threshold
  MaxLimitCrossed : Outport  OutDataTypeStr=boolean
  MinLimitCrossed : Outport  Port=2  OutDataTypeStr=boolean
  ErrorCode : Outport  Port=3  OutDataTypeStr=int64
  wires:
  Enable/disable/1 -> If/1
  If/2 -> Enabled Subsystem/Action
  If/1 -> Enabled Subsystem1/Action
  Enabled Subsystem1/3(ErrorCode) -> [If_Errorcode]
  Enabled Subsystem/2(ErrorCode) -> [Else_Errorcode]
  Enabled Subsystem/1("MaxLimitCrossed ") -> [Else_MaxLimitCrossed]
  [If_MaxLimitCrossed] -> Switch/1
  [If_Errorcode] -> Switch3/1
  [Else_Errorcode] -> Switch3/3
  Enabled Subsystem1/1(MaxLimitCrossed) -> [If_MaxLimitCrossed]
  Switch/1 -> MaxLimitCrossed/1
  [Else_MaxLimitCrossed] -> Switch/3
  Enable/disable1/1 -> Switch3/2, Switch1/2, Switch/2
  "Input "/1 -> Enabled Subsystem1/1("Input ")
  UpperTrhd/1 -> Enabled Subsystem1/2(UpperTrhd)
  LowerTrhd/1 -> Enabled Subsystem1/3(LowerTrhd)
  AbsHyst/1 -> Enabled Subsystem1/5(AbsHyst)
  RelHyst/1 -> Enabled Subsystem1/6(RelHyst)
  HystSelection/1 -> Enabled Subsystem1/4(HystSelection)
  Enabled Subsystem1/2(MinLimitCrossed) -> [If_MinLimitCrossed]
  Enabled Subsystem/3(MinLimitCrossed) -> [Else_MinLimitCrossed]
  [If_MinLimitCrossed] -> Switch1/1
  [Else_MinLimitCrossed] -> Switch1/3
  Switch1/1 -> MinLimitCrossed/1
  Switch3/1 -> ErrorCode/1

== system ESSLibrary/Comparator/Basic alarm ver2.0/Enabled Subsystem ==
  Action Port : ActionPort
  Constant3 : Constant  Value=0  OutDataTypeStr=boolean  SampleTime=-1
  "MaxLimitCrossed " : Outport
  ErrorCode : Outport  Port=2
  MinLimitCrossed : Outport  Port=3
  wires:
  Constant3/1 -> ErrorCode/1, MinLimitCrossed/1, "MaxLimitCrossed "/1

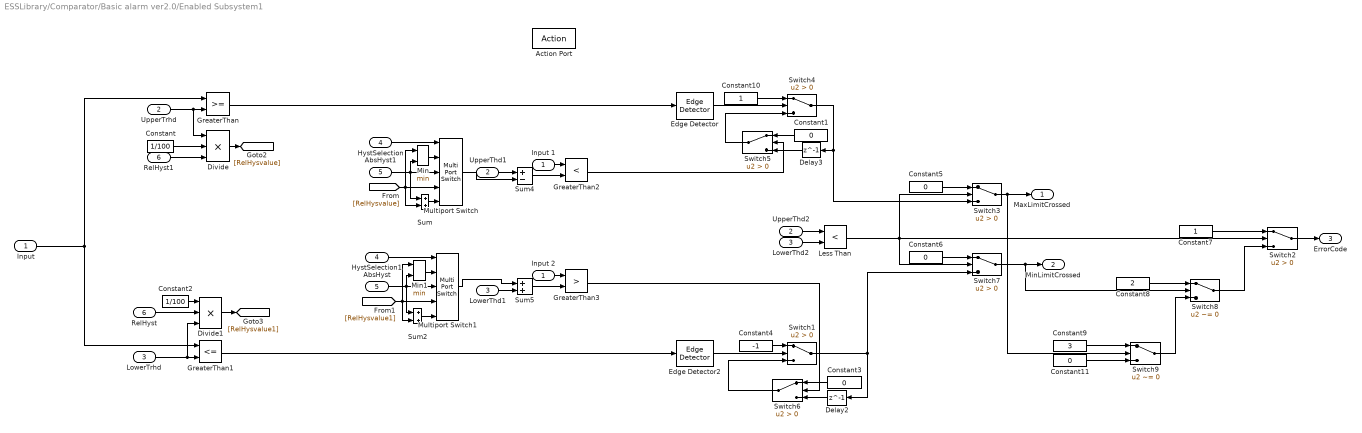
== system ESSLibrary/Comparator/Basic alarm ver2.0/Enabled Subsystem1 ==
  "Input " : Inport
  UpperTrhd : Inport  Port=2
  LowerTrhd : Inport  Port=3
  HystSelection : Inport  Port=4
  AbsHyst : Inport  Port=5
  RelHyst : Inport  Port=6
  Action Port : ActionPort
  AbsHyst1 : InportShadow  Port=5
  Constant : Constant  Value=1/100  SampleTime=-1
  Constant1 : Constant  Value=0  OutDataTypeStr=int8  SampleTime=-1
  Constant10 : Constant  OutDataTypeStr=int8  SampleTime=-1
  Constant11 : Constant  Value=0  OutDataTypeStr=int64  SampleTime=-1
  Constant2 : Constant  Value=1/100  SampleTime=-1
  Constant3 : Constant  Value=0  OutDataTypeStr=int8  SampleTime=-1
  Constant4 : Constant  Value=-1  OutDataTypeStr=int8  SampleTime=-1
  Constant5 : Constant  Value=0  OutDataTypeStr=boolean  SampleTime=-1
  Constant6 : Constant  Value=0  OutDataTypeStr=boolean  SampleTime=-1
  Constant7 : Constant  OutDataTypeStr=int64  SampleTime=-1
  Constant8 : Constant  Value=2  OutDataTypeStr=int64  SampleTime=-1
  Constant9 : Constant  Value=3  OutDataTypeStr=int64  SampleTime=-1
  Delay2 : Delay  DelayLength=1  InitialCondition=0
  Delay3 : Delay  DelayLength=1  InitialCondition=0
  Divide : Product  Inputs=***
  Divide1 : Product  Inputs=***
  Edge Detector : powerlib_meascontrol/Logic/Edge Detector  model=Rising  ic=0  Ts=-1
      settings: SourceProductBaseCode=PS
  Edge Detector2 : powerlib_meascontrol/Logic/Edge Detector  model=Rising  ic=0  Ts=-1
      settings: SourceProductBaseCode=PS
  GreaterThan : RelationalOperator  OutDataTypeStr=boolean  RndMeth=Simplest
  GreaterThan1 : RelationalOperator  Operator=<=  OutDataTypeStr=boolean  RndMeth=Simplest
  GreaterThan2 : RelationalOperator  Operator=<  OutDataTypeStr=boolean  RndMeth=Simplest
  GreaterThan3 : RelationalOperator  Operator=>  OutDataTypeStr=boolean  RndMeth=Simplest
  HystSelection1 : InportShadow  Port=4
  Input 1 : InportShadow
  Input 2 : InportShadow
  Less Than : RelationalOperator  Operator=<  OutDataTypeStr=boolean  RndMeth=Simplest
  LowerThd1 : InportShadow  Port=3
  LowerThd2 : InportShadow  Port=3
  Min : MinMax  Inputs=2
  Min1 : MinMax  Inputs=2
  Multiport Switch : MultiPortSwitch  Inputs=4
  Multiport Switch1 : MultiPortSwitch  Inputs=4
  RelHyst1 : InportShadow  Port=6
  Sum : Sum
  Sum2 : Sum
  Sum4 : Sum  Inputs=+-
  Sum5 : Sum
  Switch{1..7} (7 alike) : Switch  Criteria=u2 > Threshold
  Switch8 : Switch  Criteria=u2 ~= 0
  Switch9 : Switch  Criteria=u2 ~= 0
  UpperThd1 : InportShadow  Port=2
  UpperThd2 : InportShadow  Port=2
  MaxLimitCrossed : Outport
  MinLimitCrossed : Outport  Port=2
  ErrorCode : Outport  Port=3  OutDataTypeStr=int64
  wires:
  Constant4/1 -> Switch1/1
  GreaterThan/1 -> Edge Detector/1
  "Input "/1 -> GreaterThan/1, GreaterThan1/1
  UpperTrhd/1 -> Divide/1, GreaterThan/2
  LowerTrhd/1 -> Divide1/3, GreaterThan1/2
  HystSelection/1 -> Multiport Switch/1
  AbsHyst1/1 -> Min/2, Sum/1, Multiport Switch/3
  [RelHysvalue] -> Min/1, Sum/2, Multiport Switch/4
  Sum/1 -> Multiport Switch/5
  Divide/1 -> [RelHysvalue]
  Min/1 -> Multiport Switch/2
  Input 1/1 -> GreaterThan2/1
  Constant10/1 -> Switch4/1
  Edge Detector/1 -> Switch4/2
  Switch5/1 -> Switch4/3
  Switch4/1 -> Switch3/3, Delay3/1
  Constant/1 -> Divide/2
  RelHyst1/1 -> Divide/3
  RelHyst/1 -> Divide1/2
  Constant2/1 -> Divide1/1
  Divide1/1 -> [RelHysvalue1]
  HystSelection1/1 -> Multiport Switch1/1
  Min1/1 -> Multiport Switch1/2
  AbsHyst/1 -> Sum2/1, Min1/2, Multiport Switch1/3
  [RelHysvalue1] -> Sum2/2, Multiport Switch1/4, Min1/1
  Sum2/1 -> Multiport Switch1/5
  Input 2/1 -> GreaterThan3/1
  GreaterThan1/1 -> Edge Detector2/1
  Edge Detector2/1 -> Switch1/2
  Switch6/1 -> Switch1/3
  GreaterThan3/1 -> Switch6/2
  Sum4/1 -> GreaterThan2/2
  Multiport Switch/1 -> Sum4/2
  UpperThd1/1 -> Sum4/1
  Sum5/1 -> GreaterThan3/2
  Multiport Switch1/1 -> Sum5/1
  LowerThd1/1 -> Sum5/2
  GreaterThan2/1 -> Switch5/2
  Constant1/1 -> Switch5/1
  Constant3/1 -> Switch6/1
  Delay3/1 -> Switch5/3
  Delay2/1 -> Switch6/3
  Switch3/1 -> Switch9/2, MaxLimitCrossed/1
  Less Than/1 -> Switch2/2, Switch3/2, Switch7/2
  Constant5/1 -> Switch3/1
  Switch1/1 -> Switch7/3, Delay2/1
  Constant6/1 -> Switch7/1
  Switch7/1 -> Switch8/2, MinLimitCrossed/1
  Switch8/1 -> Switch2/3
  Constant7/1 -> Switch2/1
  Switch2/1 -> ErrorCode/1
  LowerThd2/1 -> Less Than/2
  UpperThd2/1 -> Less Than/1
  Constant8/1 -> Switch8/1
  Constant9/1 -> Switch9/1
  Constant11/1 -> Switch9/3
  Switch9/1 -> Switch8/3

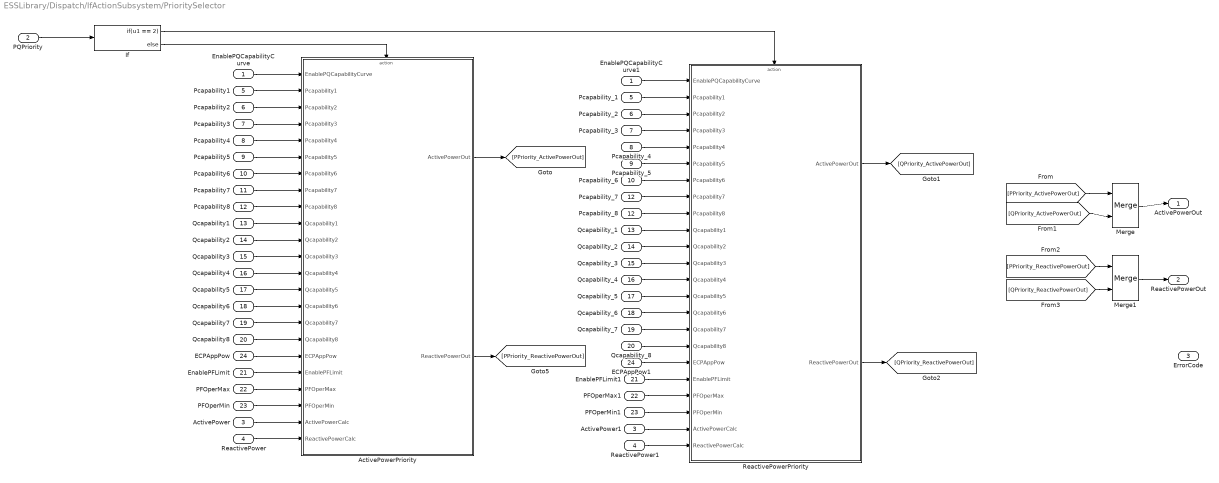
== system ESSLibrary/Dispatch/IfActionSubsystem/PrioritySelector ==
  EnablePQCapabilityCurve : Inport  OutDataTypeStr=boolean
  PQPriority : Inport  Port=2
  ActivePower : Inport  Port=3
  ReactivePower : Inport  Port=4
  Pcapability1 : Inport  Port=5
  Pcapability2 : Inport  Port=6
  Pcapability3 : Inport  Port=7
  Pcapability4 : Inport  Port=8
  Pcapability5 : Inport  Port=9
  Pcapability6 : Inport  Port=10
  Pcapability7 : Inport  Port=11
  Pcapability8 : Inport  Port=12
  Qcapability1 : Inport  Port=13
  Qcapability2 : Inport  Port=14
  Qcapability3 : Inport  Port=15
  Qcapability4 : Inport  Port=16
  Qcapability5 : Inport  Port=17
  Qcapability6 : Inport  Port=18
  Qcapability7 : Inport  Port=19
  Qcapability8 : Inport  Port=20
  EnablePFLimit : Inport  Port=21
  PFOperMax : Inport  Port=22
  PFOperMin : Inport  Port=23
  ECPAppPow : Inport  Port=24
  ActivePower1 : InportShadow  Port=3
  ActivePowerPriority : Subsystem  TreatAsAtomicUnit=on
  ECPAppPow1 : InportShadow  Port=24
  EnablePFLimit1 : InportShadow  Port=21
  EnablePQCapabilityCurve1 : InportShadow  OutDataTypeStr=boolean
  If : If  IfExpression=u1 == 2
  Merge : Merge
  Merge1 : Merge
  PFOperMax1 : InportShadow  Port=22
  PFOperMin1 : InportShadow  Port=23
  Pcapability_1 : InportShadow  Port=5
  Pcapability_2 : InportShadow  Port=6
  Pcapability_3 : InportShadow  Port=7
  Pcapability_4 : InportShadow  Port=8
  Pcapability_5 : InportShadow  Port=9
  Pcapability_6 : InportShadow  Port=10
  Pcapability_7 : InportShadow  Port=12
  Pcapability_8 : InportShadow  Port=12
  Qcapability_1 : InportShadow  Port=13
  Qcapability_2 : InportShadow  Port=14
  Qcapability_3 : InportShadow  Port=15
  Qcapability_4 : InportShadow  Port=16
  Qcapability_5 : InportShadow  Port=17
  Qcapability_6 : InportShadow  Port=18
  Qcapability_7 : InportShadow  Port=19
  Qcapability_8 : InportShadow  Port=20
  ReactivePower1 : InportShadow  Port=4
  ReactivePowerPriority : Subsystem  TreatAsAtomicUnit=on
  ActivePowerOut : Outport
  ReactivePowerOut : Outport  Port=2
  ErrorCode : Outport  Port=3
  wires:
  PQPriority/1 -> If/1
  Merge/1 -> ActivePowerOut/1
  Merge1/1 -> ReactivePowerOut/1
  If/2 -> ActivePowerPriority/Action
  If/1 -> ReactivePowerPriority/Action
  ? -> ErrorCode/1
  EnablePQCapabilityCurve/1 -> ActivePowerPriority/1("EnablePQCapabilityCurve ")
  Pcapability1/1 -> ActivePowerPriority/2(Pcapability1)
  Pcapability2/1 -> ActivePowerPriority/3(Pcapability2)
  Pcapability3/1 -> ActivePowerPriority/4(Pcapability3)
  Pcapability4/1 -> ActivePowerPriority/5(Pcapability4)
  Pcapability5/1 -> ActivePowerPriority/6(Pcapability5)
  Pcapability6/1 -> ActivePowerPriority/7(Pcapability6)
  Pcapability7/1 -> ActivePowerPriority/8(Pcapability7)
  Pcapability8/1 -> ActivePowerPriority/9(Pcapability8)
  Qcapability1/1 -> ActivePowerPriority/10(Qcapability1)
  Qcapability2/1 -> ActivePowerPriority/11(Qcapability2)
  Qcapability3/1 -> ActivePowerPriority/12(Qcapability3)
  Qcapability4/1 -> ActivePowerPriority/13(Qcapability4)
  Qcapability5/1 -> ActivePowerPriority/14(Qcapability5)
  Qcapability6/1 -> ActivePowerPriority/15(Qcapability6)
  Qcapability7/1 -> ActivePowerPriority/16(Qcapability7)
  Qcapability8/1 -> ActivePowerPriority/17(Qcapability8)
  EnablePFLimit/1 -> ActivePowerPriority/19(EnablePFLimit)
  PFOperMax/1 -> ActivePowerPriority/20(PFOperMax)
  PFOperMin/1 -> ActivePowerPriority/21(PFOperMin)
  ActivePower/1 -> ActivePowerPriority/22(ActivePowerCalc)
  ReactivePower/1 -> ActivePowerPriority/23(ReactivePowerCalc)
  EnablePQCapabilityCurve1/1 -> ReactivePowerPriority/1("EnablePQCapabilityCurve ")
  Qcapability_8/1 -> ReactivePowerPriority/17(Qcapability8)
  Qcapability_7/1 -> ReactivePowerPriority/16(Qcapability7)
  Qcapability_6/1 -> ReactivePowerPriority/15(Qcapability6)
  Qcapability_5/1 -> ReactivePowerPriority/14(Qcapability5)
  Qcapability_4/1 -> ReactivePowerPriority/13(Qcapability4)
  Qcapability_3/1 -> ReactivePowerPriority/12(Qcapability3)
  Qcapability_2/1 -> ReactivePowerPriority/11(Qcapability2)
  Qcapability_1/1 -> ReactivePowerPriority/10(Qcapability1)
  Pcapability_8/1 -> ReactivePowerPriority/9(Pcapability8)
  Pcapability_7/1 -> ReactivePowerPriority/8(Pcapability7)
  Pcapability_6/1 -> ReactivePowerPriority/7(Pcapability6)
  Pcapability_5/1 -> ReactivePowerPriority/6(Pcapability5)
  Pcapability_4/1 -> ReactivePowerPriority/5(Pcapability4)
  Pcapability_3/1 -> ReactivePowerPriority/4(Pcapability3)
  Pcapability_2/1 -> ReactivePowerPriority/3(Pcapability2)
  Pcapability_1/1 -> ReactivePowerPriority/2(Pcapability1)
  EnablePFLimit1/1 -> ReactivePowerPriority/19(EnablePFLimit)
  PFOperMin1/1 -> ReactivePowerPriority/21(PFOperMin)
  PFOperMax1/1 -> ReactivePowerPriority/20(PFOperMax)
  ActivePower1/1 -> ReactivePowerPriority/22(ActivePowerCalc)
  ReactivePower1/1 -> ReactivePowerPriority/23(ReactivePowerCalc)
  ECPAppPow/1 -> ActivePowerPriority/18(ECPAppPow)
  ECPAppPow1/1 -> ReactivePowerPriority/18(ECPAppPow)
  ActivePowerPriority/2(ReactivePowerOut) -> [PPriority_ReactivePowerOut]
  ActivePowerPriority/1(ActivePowerOut) -> [PPriority_ActivePowerOut]
  ReactivePowerPriority/2(ReactivePowerOut) -> [QPriority_ReactivePowerOut]
  ReactivePowerPriority/1(ActivePowerOut) -> [QPriority_ActivePowerOut]
  [PPriority_ActivePowerOut] -> Merge/1
  [QPriority_ActivePowerOut] -> Merge/2
  [PPriority_ReactivePowerOut] -> Merge1/1
  [QPriority_ReactivePowerOut] -> Merge1/2
